simulink library "Lib_Analytic"  (R2019b)
settings: Solver=VariableStepAuto  StartTime=0.0  StopTime=10.0  RelTol=1e-3
undefined symbols (not defined in the file): SJac_Per_M, SNR_DX_M, SNR_IC_M, SNR_Mn_M, SNR_Mx_M
libraries: simulink x2
(part 1 of 2)
settings Model: Creator=sbianco1  LastModifiedBy=sbianco1

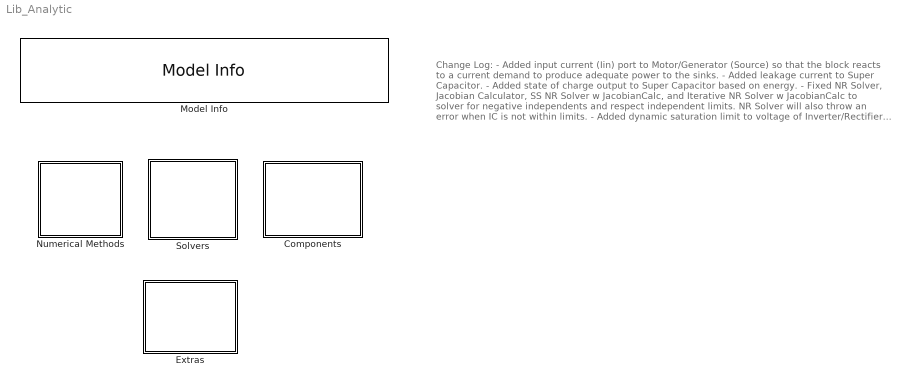
== system Lib_Analytic ==
  note: Change Log:
      | - Added input current (Iin) port to Motor/Generator (Source) so that the block reacts to a current demand to produce adequate power to the sinks.
      | - Added leakage current to Super Capacitor.
      | - Added state of charge output to Super Capacitor based on energy.
      | - Fixed NR Solver, Jacobian Calculator, SS NR Solver w JacobianCalc, and Iterative NR Solver w JacobianCalc to solver for negative independents and respect independent limits. NR Solver will also throw an error when IC is not within limits.
      | - Added dynamic saturation limit to voltage of Inverter/Rectifier (Sink). The back EMF produced by the rotation of the motor limits the voltage output to the motor. It cannot go higher than the input voltage. This limits the speed of the motor.
      | - Added subsystem in multiple blocks inside Components (Analytical) to address calculation problems when Vin = 0.
      | - Created a temperature block.
  Components : Subsystem
  Extras : Subsystem
  Model Info : simulink/Model-Wide Utilities/Model Info  Frame=on  DisplayStringWithTags=|  HorizontalTextAlignment=Left  LeftAlignmentValue=0.02
      | Created by: Santino Bianco and Mark Bell with references from Jeff Chapman.
      | Version: %<ModelVersion>
  Numerical Methods : Subsystem
  Solvers : Subsystem

== system Lib_Analytic/Components ==
  Active Resistor : Subsystem  ClipboardFcn=|  mask(Active Resistor){}
      | Active Resistor
      | Version: %<LibraryVersion>
      mask help: This block changes its resistance (R) based on a power command (Pset) to produce a current demand (Iin).
      settings: AttributesFormatString=|
      | Active Resistor
      | Version: %<LibraryVersion>
  Cable : Subsystem  mask(Cable){R_c=0.2, I_IC=0}
      mask prompts: R_c "R_c - Resistance, Ohm"; I_IC "I_IC - Initial Current, A"
      mask help: This block models a cable with resistive line effects.
      settings: AttributesFormatString=|
      | Cable
      | Version: %<LibraryVersion>
  Current Junction : Subsystem  mask(Current Junction){}
      mask help: This block adds a vector of input currents (I).
      settings: AttributesFormatString=|
      | Current Junction
      | Version: %<LibraryVersion>
      mask DialogControl Control2 Prompt: Note: There is no limit to the number of multiplexed currents.
  DC-DC Converter : Subsystem  mask(DC-DC Converter){X_Vin_VoltageVec_M=[0 100 1000 5000], Y_Iout_CurrentVec_M=[0 10 100 150], T_C_EffArray_M=0.98*ones(4,4)}
      mask prompts: X_Vin_VoltageVec_M "X_Vin_VoltageVec_M - Efficiency Table Voltage Vector (X-axis)(nx1)"; Y_Iout_CurrentVec_M "Y_Iout_CurrentVec_M - Efficiency Table Current Vector (Y-axis)(mx1)"; T_C_EffArray_M "T_C_EffArray_M - Efficiency Table Values (Eff = f(i, V)(nxm)"
      mask help: This block models the power flow through a DC-DC converter using a user specified efficiency table. The output voltage (Vout) can also be set using variable Vset.
      settings: AttributesFormatString=|
      | DC-DC Converter
      | Version: %<LibraryVersion>
  Inverter/Rectifier (Sink) : Subsystem  mask(Inverter/Rectifier - Sink){X_C_VoltageVec_M=[0 100 1000 5000], Y_C_CurrentVec_M=[0 10 100 150], T_C_EffArray_M=.90*ones(4,4), K_e=0.0503}
      mask prompts: X_C_VoltageVec_M "X_C_VoltageVec_M - Efficiency Table Voltage Vector (X-axis)(nx1)"; Y_C_CurrentVec_M "Y_C_CurrentVec_M - Efficiency Table Current Vector (Y-axis)(mx1)"; T_C_EffArray_M "T_C_EffArray_M - Efficiency Table Values (Eff = f(i, V)(nxm)"; K_e "K_e - Back EMF Constant, V/RPM"
      mask help: This block models an inverter/rectifier for use as a power sink. The power through the inverter/rectifier is modified by a user-input efficiency table.
      settings: AttributesFormatString=|
      | Inverter/Rectifier (Sink)
      | Version: %<LibraryVersion>
  Inverter/Rectifier (Source) : Subsystem  mask(Inverter/Rectifier - Source){X_Vout_VoltageVec_M=[0 100 1000 5000], Y_Iin_CurrentVec_M=[0 10 100 150], T_C_EffArray_M=.90*ones(4,4)}
      mask prompts: X_Vout_VoltageVec_M "X_Vout_VoltageVec_M - Efficiency Table Voltage Vector (X-axis)(nx1)"; Y_Iin_CurrentVec_M "Y_Iin_CurrentVec_M - Efficiency Table Current Vector (Y-axis)(mx1)"; T_C_EffArray_M "T_C_EffArray_M - Efficiency Table Values (Eff = f(i, V)(nxm)"
      mask help: This block models an inverter/rectifier for use as a power source. The power through the inverter/rectifier is modified by a user-input efficiency table.
      settings: AttributesFormatString=|
      | Inverter/Rectifier (Source)
      | Version: %<LibraryVersion>
  Mechanical Shaft : Subsystem  mask(Mechanical Shaft){J=0.01, B=0.001, N_IC=0}
      mask prompts: J "J - Inertia, lb-ft-s^2"; B "B - Damping, lb-ft-s"; N_IC "N_IC - Initial Speed, RPM"
      mask help: This block models a mechanical shaft with inertia and damping effects.
      settings: AttributesFormatString=|
      | Mechanical Shaft
      | Version: %<LibraryVersion>
  Motor/Generator (Sink) : Subsystem  mask(Motor/Generator - Sink){X_C_SpeedVec_M=[0 100 1000 5000], Y_C_TorqueVec_M=[0 10 100 150], T_C_EffArray_M=0.99*ones(4,4)}
      mask prompts: X_C_SpeedVec_M "X_C_SpeedVec_M - Efficiency Table Speed Vector (X-axis)(nx1)"; Y_C_TorqueVec_M "Y_C_TorqueVec_M - Efficiency Table Torque Vector (Y-axis)(mx1)"; T_C_EffArray_M "T_C_EffArray_M - Efficiency Table Values (Eff = f(i, V)(nxm)"
      mask help: This block models an motor/generator for use as a power sink. The power through the motor/generator is modified by a user-input efficiency table.
      settings: AttributesFormatString=|
      | Motor/Generator (Sink)
      | Version: %<LibraryVersion>
  Motor/Generator (Source) : Subsystem  mask(Motor/Generator - Source){X_C_SpeedVec_M=[0 100 1000 5000], Y_C_TorqueVec_M=[0 10 100 150], T_C_EffArray_M=0.99*ones(4,4), K_e=0.0503, K_t=0.0503}
      mask prompts: X_C_SpeedVec_M "X_C_SpeedVec_M - Efficiency Table Speed Vector (X-axis)(nx1)"; Y_C_TorqueVec_M "Y_C_TorqueVec_M - Efficiency Table Torque Vector (Y-axis)(mx1)"; T_C_EffArray_M "T_C_EffArray_M - Efficiency Table Values (Eff = f(i, V)(nxm)"; K_e "K_e - Back EMF Constant, V/RPM"; K_t "K_t - Torque Constant, lbf-ft/A"
      mask help: This block models an motor/generator for use as a power source. The power through the motor/generator is modified by a user-input efficiency table.
      settings: AttributesFormatString=|
      | Motor/Generator (Source)
      | Version: %<LibraryVersion>
  Super Capacitor : Subsystem  mask(Super Capacitor){C=130, ESR=0.02, ILeak=0, TSE=69, Iout_IC=0, V_IC=150}
      mask prompts: C "C - Capacitance, H"; ESR "ESR - Equivilent Series Resistance, Ohm"; ILeak "ILeak - Leakage Current per Time Step, A"; TSE "TSE - Max Stored Energy, W-h"; Iout_IC "Iout_IC - Initial Output Current, A"; V_IC "V_IC - Initial Voltage, V"
      mask help: This block models a capacitor with equivilent series resistive (ESR) effects.
      settings: AttributesFormatString=|
      | Super Capacitor
      | Version: %<LibraryVersion>

== system Lib_Analytic/Extras ==
  Exergy : Subsystem  mask(Exergy){m=0, Cp=0}
      mask prompts: m "m - Mass, slug"; Cp "Cp - Specific Heat, Btu/degF"
      mask help: This block calculated the exergy of a component given the component's generated heat, mass, material specific heat, and chnage in ambient temperature from sea level static (SLS).
      settings: AttributesFormatString=|
      | Exergy
      | Version: %<LibraryVersion>
  Temperature : Subsystem  mask(Temperature){m=0, Cp=0}
      mask prompts: m "m - Mass, lbm"; Cp "Cp - Specific Heat, Btu/(lbm-degF)"
      mask help: This block converts a heat output (Heat) from an electrical component to a temperature (Temp) using the ambient temperature (Ambient Temp) and possibly a change in ambient temperature from sea-level static (dTamb) as inputs. A mass in units of pound-mass and a specific heat in units of Btu/(lbm-degF) must be specified.
      settings: AttributesFormatString=|
      | Temperature
      | Version: %<LibraryVersion>
      mask DialogControl Container3 Prompt: Physical Parameters

== system Lib_Analytic/Numerical Methods ==
  Jacobian Calculator : Subsystem  TreatAsAtomicUnit=on  mask(T-MATS: Jacobian Calculator Library Block){N_Per_M=SJac_Per_M}
      mask prompts: N_Per_M "N_Per_M - Perturbations (nxm)"
      mask help:
      | The Jacobian Calculator block calculates the Jabobian of the system by perturbing the system around an initial point and calculating the gradient for each perturbation. This module will run once on start up and then again only if the reset is pressed.
      | Below: n (rows) is the number of times each independent will be perturbed and m (columns) is the number of inputs.
      settings: AttributesFormatString=|
      | Jacobian Calculator
      | Version: %<LibraryVersion>
      mask Help: web(which('NumMthd_TMATS_JC.html'),'-helpbrowser')
  Newton Raphson Solver : Subsystem  TreatAsAtomicUnit=on  mask(T-MATS: Newton Raphson Solver Library Block){NR_IC_M=SNR_IC_M./abs(SNR_IC_M), NR_dx_Lim_M=SNR_DX_M, NR_Mx_Lim_M=SNR_Mx_M./abs(SNR_IC_M), NR_Mn_Lim_M=SNR_Mn_M./abs(SNR_IC_M), BlkNm_M=double(gcb)}
      mask prompts: NR_IC_M "NR_IC_M - Initial Conditions of Newton Raphson (mx1)"; NR_dx_Lim_M "NR_dx_Lim_M - Newton Raphson step size limit (%) (1x1)"; NR_Mx_Lim_M "NR_Mx_Lim_M - Max limit (1x1 or mx1)"; NR_Mn_Lim_M "NR_Mn_Lim_M - Min Limit (1x1 or mx1)"; BlkNm_M "BlkNm_M - Block Name"
      mask help:
      | Newton Raphson Solver:
      |
      | x(n+1) = x(n) - inverse(f'(x(n)))*f(x(n))
      |
      | Note:
      | inverse(f'(x(n))) is an m x m matrix and f(x(n)) is an m x 1 matrix
      | where m is the length of the initial conditions matrix and number of system independents.
      mask init:
      | if isequal(size(NR_Mx_Lim_M),size(NR_IC_M))
      | elseif isequal(size(NR_Mx_Lim_M),size(1))
      | else
      |     warning('NR_Mx_Lim_M must be the same size as NR_IC_M or a constant')
      | end
      | 
      | if isequal(size(NR_Mn_Lim_M),size(NR_IC_M))
      | elseif isequal(size(NR_Mn_Lim_M),size(1))
      | else
      |     warning('NR_Mn_Lim_M must be the same size as NR_IC_M or a constant')
      | end
      settings: AttributesFormatString=|
      | Newton Raphson Solver
      | Version: %<LibraryVersion>
      mask Help: web(which('NumMthd_TMATS_NRS.html'),'-helpbrowser')

== system Lib_Analytic/Solvers ==
  Iterative NR Solver w JacobianCalc : Subsystem  mask(T-MATS: Iterative NR Solver w Jacobian Calc Library Block){SJac_Per_M=0.01*ones(2,2), SNR_IC_M=[-4;1], SNR_DX_M=5, SNR_Mx_M=100000, SNR_Mn_M=-100000, SJacobianAttempts_M=20, Cond_Limits_M=0.0001}
      mask prompts: SJac_Per_M "SJac_Per_M - Jacobian Perturbation size (frac) (nxm)"; SNR_IC_M "SNR_IC_M - Newton Raphson Initial Conditions (mx1)"; SNR_DX_M "SNR_DX_M - Newton Raphson step size limiter (%) (1x1)"; SNR_Mx_M "SNR_Mx_M - Newton Raphson max limit (1x1 or mx1)"; SNR_Mn_M "SNR_Mn_M - Newton Raphson min limit (1x1 or mx1)"; SJacobianAttempts_M "SJacobianAttempts_M - Newton Raphson attempts before the Jacobian recalculation (1x1)"; Cond_Limits_M "Cond_Limits_M - Iteration Conditions Limits (mx1 or 1x1)"
      mask help:
      | The Iterative Newton Raphson Solver with Jacobian Calculator block will
      | supply the inputs to iteratively drive the outputs of a system to zero.
      |
      | This will be performed in three steps.
      | 1) Jabobian calculator sends Perturbations to the plant then calculates the plant
      | Jacboian based on the system response
      | 2) The Newton Raphson will use the inverse of the Jacobian to iteratively step the
      | system toward solution.
      | 3) Once the solution has satisfied the conditions the Newton Raphson is shut off.
      |
      | This module is designed for dynamic systems and should be paired with
      | a "do... while" block in Simulink. The "do...while" block and this module
      | should both be located in the same subsystem as the plant that is to be solved for.
      mask init:
      | if isequal(size(SNR_Mx_M),size(SNR_IC_M))
      | elseif isequal(size(SNR_Mx_M),[1 1])
      | else
      |     disp('NR_Mx_Lim_M must be the same size as NR_IC_M or a constant')
      | end
      | 
      | if isequal(size(SNR_Mn_M),size(SNR_IC_M))
      | elseif isequal(size(SNR_Mn_M),[1 1])
      | else
      |     disp('NR_Mn_Lim_M must be the same size as NR_IC_M or a constant')
      | end
      settings: AttributesFormatString=|
      | Iterative NR Solver w JacobianCalc
      | Version: %<LibraryVersion>
      mask Help: web(which('Solver_TMATS_INRSwJC.html'),'-helpbrowser')
  SS NR Solver w JacobianCalc : Subsystem  mask(T-MATS: SS NR Solver w Jacobian Calc Library Block){SJac_Per_M=0.01*ones(2,2), SNR_IC_M=[-4;5], SNR_DX_M=5, SNR_Mx_M=100000, SNR_Mn_M=-100000, SJacobianAttempts_M=20, Cond_Limits_M=0.0001}
      mask prompts: SJac_Per_M "SJac_Per_M - Jacobian Perturbation size (frac)(nxm)"; SNR_IC_M "SNR_IC_M - Newton Raphson Initial Conditions (mx1)"; SNR_DX_M "SNR_DX_M - Newton Raphson step size limit (%) (1x1)"; SNR_Mx_M "SNR_Mx_M - Newton Raphson max limit (1x1 or mx1)"; SNR_Mn_M "SNR_Mn_M - Newton Raphson min limit (1x1 or mx1)"; SJacobianAttempts_M "SJacobianAttempts_M - Newton Raphson attempts before the Jacobian recalculation (1x1)"; Cond_Limits_M "Cond_Limits_M - Iteration Conditions Limits (mx1 or 1x1)"
      mask help:
      | The Steady State Newton Raphson Solver with Jacobian Calculator block will
      | supply the inputs to iteratively drive the outputs of a system to zero.
      |
      | This will be performed in three steps.
      | 1) Jabobian calculator sends Perturbations to the plant then calculates the plant
      | Jacboian based on the system response
      | 2) The Newton Raphson will use the inverse of the Jacobian to iteratively step the
      | system toward solution.
      | 3) Once the solution has satisfied the conditions the Newton Raphson is shut off.
      |
      | Simulation run time length should be selected as to give the Newton Raphson solver adequate time to develop a solution.
      mask init: same as Lib_Analytic/Solvers/Iterative NR Solver w JacobianCalc
      settings: AttributesFormatString=|
      | SS NR Solver w JacobianCalc
      | Version: %<LibraryVersion>
      mask Help: web(which('Solver_TMATS_SSNRwJC.html'),'-helpbrowser')

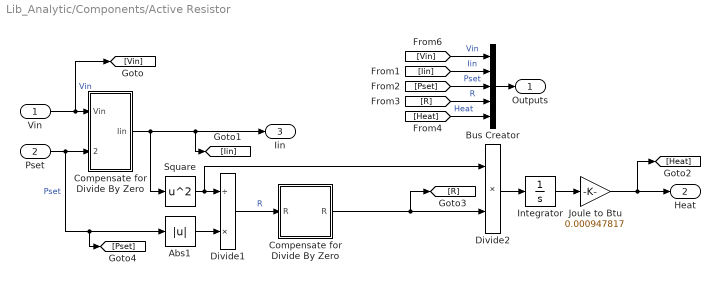
== system Lib_Analytic/Components/Active Resistor ==
  Vin : Inport
  "Pset " : Inport  Port=2
  Abs1 : Abs
  Bus Creator : BusCreator  Inputs=5
  Compensate for Divide By Zero : Subsystem
  "Compensate for Divide By Zero " : Subsystem
  Divide1 : Product  Inputs=/*
  Divide2 : Product  Inputs=**
  Integrator : Integrator
  Joule to Btu : Gain  Gain=0.000947817
  Square : Math  Operator=square  SignedPower=off  SaturateOnIntegerOverflow=on
  Outputs : Outport
  Heat : Outport  Port=2
  Iin : Outport  Port=3
  wires:
  Bus Creator/1 -> Outputs/1
  Divide1/1 -> Compensate for Divide By Zero/1(R)  "R"
  Square/1 -> Divide2/1, Divide1/1
  "Pset "/1 -> "Compensate for Divide By Zero "/2(Pset), [Pset], Abs1/1  "Pset"
  Vin/1 -> [Vin], "Compensate for Divide By Zero "/1(Vin)  "Vin"
  Divide2/1 -> Integrator/1
  Integrator/1 -> Joule to Btu/1
  Joule to Btu/1 -> [Heat], Heat/1
  [Vin] -> Bus Creator/1  "Vin"
  [Iin] -> Bus Creator/2  "Iin"
  [Pset] -> Bus Creator/3  "Pset"
  [R] -> Bus Creator/4  "R"
  [Heat] -> Bus Creator/5  "Heat"
  Abs1/1 -> Divide1/2
  Compensate for Divide By Zero/1("R ") -> [R], Divide2/2
  "Compensate for Divide By Zero "/1(Iin) -> [Iin], Iin/1, Square/1

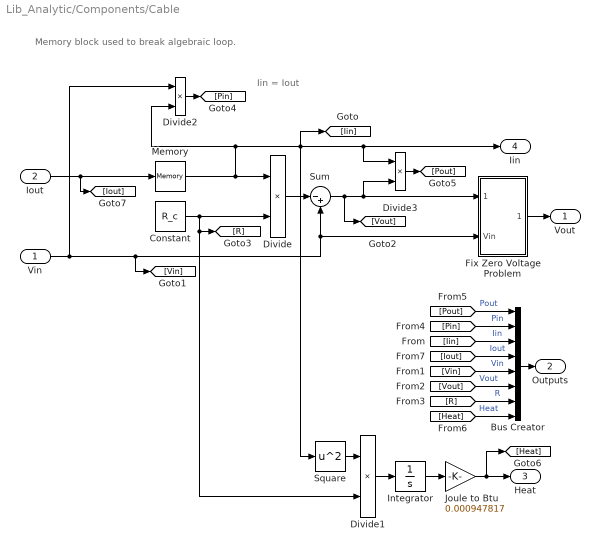
== system Lib_Analytic/Components/Cable ==
  note: Iin = Iout
  note: Memory block used to break algebraic loop.
  Vin : Inport
  Iout : Inport  Port=2
  Bus Creator : BusCreator  Inputs=8
  Constant : Constant  Value=R_c
  Divide{,1..3} (4 alike) : Product  Inputs=**
  Fix Zero Voltage Problem : Subsystem
  Integrator : Integrator
  Joule to Btu : Gain  Gain=0.000947817
  Memory : Memory  InitialCondition=I_IC
  Square : Math  Operator=square  SignedPower=off  SaturateOnIntegerOverflow=on
  Sum : Sum  Inputs=|-+
  Vout : Outport
  Outputs : Outport  Port=2
  Heat : Outport  Port=3
  Iin : Outport  Port=4
  wires:
  Divide/1 -> Sum/1
  Vin/1 -> Divide2/1, Sum/2, Fix Zero Voltage Problem/2(Vin), [Vin]
  Sum/1 -> [Vout], Fix Zero Voltage Problem/1("Vout "), Divide3/2
  Memory/1 -> Square/1, Divide3/1, Iin/1, [Iin], Divide2/2, Divide/1
  Iout/1 -> [Iout], Memory/1
  [Iin] -> Bus Creator/3  "Iin"
  [Vout] -> Bus Creator/6  "Vout"
  [Vin] -> Bus Creator/5  "Vin"
  Bus Creator/1 -> Outputs/1
  [R] -> Bus Creator/7  "R"
  Constant/1 -> Divide1/2, [R], Divide/2
  Square/1 -> Divide1/1
  Divide1/1 -> Integrator/1
  Joule to Btu/1 -> [Heat], Heat/1
  Integrator/1 -> Joule to Btu/1
  [Pin] -> Bus Creator/2  "Pin"
  [Pout] -> Bus Creator/1  "Pout"
  Divide2/1 -> [Pin]
  Divide3/1 -> [Pout]
  [Heat] -> Bus Creator/8  "Heat"
  Fix Zero Voltage Problem/1(Vout) -> Vout/1
  [Iout] -> Bus Creator/4  "Iout"

== system Lib_Analytic/Components/Current Junction ==
  I : Inport
  Sum of Elements : Sum  Inputs=+
  Isum : Outport
  wires:
  I/1 -> Sum of Elements/1
  Sum of Elements/1 -> Isum/1

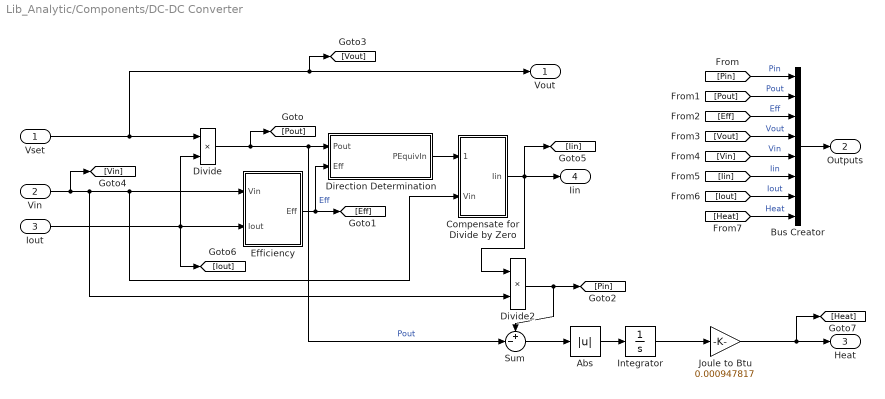
== system Lib_Analytic/Components/DC-DC Converter ==
  Vset : Inport
  Vin : Inport  Port=2
  Iout : Inport  Port=3
  Abs : Abs
  Bus Creator : BusCreator  Inputs=8
  Compensate for Divide by Zero : Subsystem
  Direction Determination : Subsystem
  Divide : Product  Inputs=**
  Divide2 : Product  Inputs=**
  Efficiency : Subsystem
  Integrator : Integrator
  Joule to Btu : Gain  Gain=0.000947817
  Sum : Sum  Inputs=+-|
  Vout : Outport
  Outputs : Outport  Port=2
  Heat : Outport  Port=3
  Iin : Outport  Port=4
  wires:
  Vset/1 -> [Vout], Vout/1, Divide/1
  Joule to Btu/1 -> [Heat], Heat/1
  Vin/1 -> [Vin], Divide2/2, Compensate for Divide by Zero/2(Vin), Efficiency/1(Vin)
  Compensate for Divide by Zero/1(Iin) -> [Iin], Divide2/1, Iin/1
  Direction Determination/1(PEquivIn) -> Compensate for Divide by Zero/1(PEquivIn)
  Efficiency/1(Eff) -> Direction Determination/2(Eff), [Eff]  "Eff"
  Divide/1 -> Sum/2, Direction Determination/1(Pout), [Pout]  "Pout"
  Bus Creator/1 -> Outputs/1
  Divide2/1 -> [Pin], Sum/1
  [Pin] -> Bus Creator/1  "Pin"
  [Pout] -> Bus Creator/2  "Pout"
  [Eff] -> Bus Creator/3  "Eff"
  [Vout] -> Bus Creator/4  "Vout"
  [Vin] -> Bus Creator/5  "Vin"
  [Iin] -> Bus Creator/6  "Iin"
  Iout/1 -> Divide/2, [Iout], Efficiency/2(Iout)
  [Iout] -> Bus Creator/7  "Iout"
  [Heat] -> Bus Creator/8  "Heat"
  Integrator/1 -> Joule to Btu/1
  Abs/1 -> Integrator/1
  Sum/1 -> Abs/1

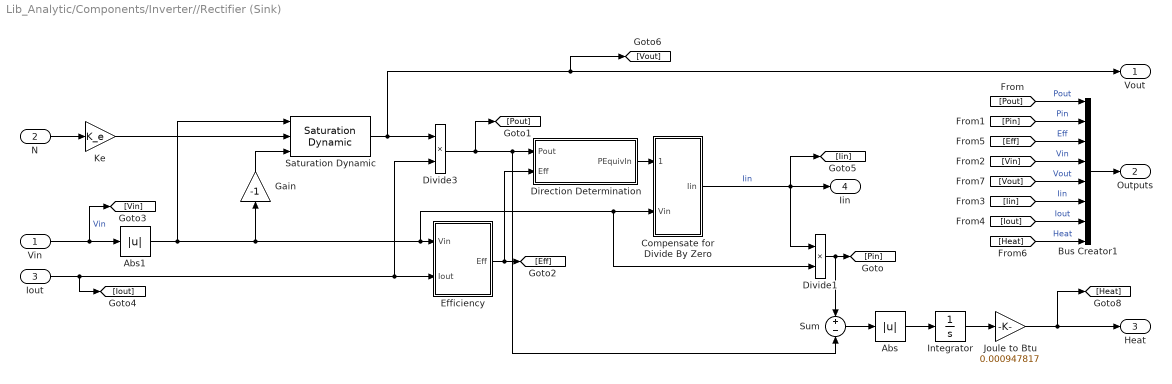
== system Lib_Analytic/Components/Inverter//Rectifier (Sink) ==
  Vin : Inport
  N : Inport  Port=2
  Iout : Inport  Port=3
  Abs : Abs
  Abs1 : Abs
  Bus Creator1 : BusCreator  Inputs=8
  Compensate for Divide By Zero : Subsystem
  Direction Determination : Subsystem
  Divide1 : Product  Inputs=**
  Divide3 : Product  Inputs=**
  Efficiency : Subsystem
  Gain : Gain  Gain=-1
  Integrator : Integrator
  Joule to Btu : Gain  Gain=0.000947817
  Ke : Gain  Gain=K_e
  Saturation Dynamic : simulink/Discontinuities/Saturation Dynamic  OutMin=[]  OutMax=[]  OutDataTypeStr=Inherit: Same as second input  OutDataType=fixdt(1, 16)  OutScaling=2^-10  DoSatur=off
  Sum : Sum  Inputs=+-
  Vout : Outport
  Outputs : Outport  Port=2
  Heat : Outport  Port=3
  Iin : Outport  Port=4
  wires:
  Iout/1 -> [Iout], Efficiency/2(Iout), Divide3/2
  Vin/1 -> [Vin], Abs1/1  "Vin"
  Divide3/1 -> Direction Determination/1(Pout), Sum/2, [Pout]
  Compensate for Divide By Zero/1(Iin) -> [Iin], Divide1/1, Iin/1  "Iin"
  Efficiency/1(Eff) -> [Eff], Direction Determination/2(Eff)
  Ke/1 -> Saturation Dynamic/2
  N/1 -> Ke/1
  [Pin] -> Bus Creator1/2  "Pin"
  [Pout] -> Bus Creator1/1  "Pout"
  [Vin] -> Bus Creator1/4  "Vin"
  [Iin] -> Bus Creator1/6  "Iin"
  Bus Creator1/1 -> Outputs/1
  [Eff] -> Bus Creator1/3  "Eff"
  [Iout] -> Bus Creator1/7  "Iout"
  Direction Determination/1(PEquivIn) -> Compensate for Divide By Zero/1(PEquivIn)
  Divide1/1 -> Sum/1, [Pin]
  [Heat] -> Bus Creator1/8  "Heat"
  [Vout] -> Bus Creator1/5  "Vout"
  Sum/1 -> Abs/1
  Abs/1 -> Integrator/1
  Integrator/1 -> Joule to Btu/1
  Joule to Btu/1 -> [Heat], Heat/1
  Saturation Dynamic/1 -> [Vout], Vout/1, Divide3/1
  Gain/1 -> Saturation Dynamic/3
  Abs1/1 -> Saturation Dynamic/1, Gain/1, Divide1/2, Compensate for Divide By Zero/2(Vin), Efficiency/1(Vin)

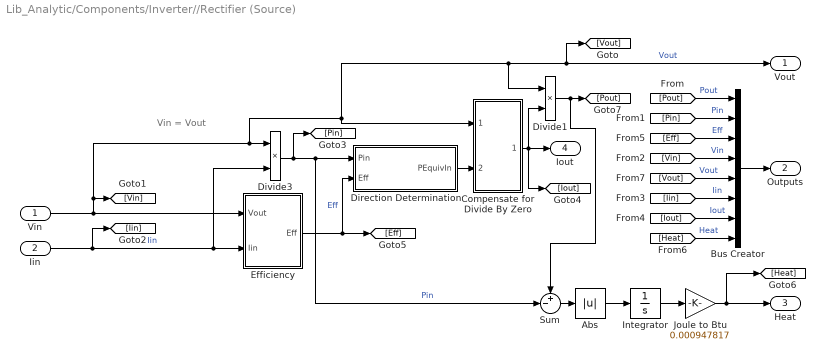
== system Lib_Analytic/Components/Inverter//Rectifier (Source) ==
  note: Vin = Vout
  Vin : Inport
  Iin : Inport  Port=2
  Abs : Abs
  Bus Creator : BusCreator  Inputs=8
  Compensate for Divide By Zero : Subsystem
  Direction Determination : Subsystem
  Divide1 : Product  Inputs=**
  Divide3 : Product  Inputs=**
  Efficiency : Subsystem
  Integrator : Integrator
  Joule to Btu : Gain  Gain=0.000947817
  Sum : Sum  Inputs=+-|
  Vout : Outport
  Outputs : Outport  Port=2
  Heat : Outport  Port=3
  Iout : Outport  Port=4
  wires:
  Vin/1 -> Efficiency/1(Vout), [Vin], Divide3/1, Compensate for Divide By Zero/1(Vout), Divide1/1, [Vout], Vout/1  "Vout"
  Efficiency/1(Eff) -> [Eff], Direction Determination/2(Eff)  "Eff"
  Compensate for Divide By Zero/1(Iout) -> Divide1/2, Iout/1, [Iout]
  Bus Creator/1 -> Outputs/1
  Divide3/1 -> [Pin], Sum/2, Direction Determination/1(Pin)  "Pin"
  Iin/1 -> [Iin], Divide3/2, Efficiency/2(Iin)  "Iin"
  Direction Determination/1(PEquivIn) -> Compensate for Divide By Zero/2(PEquivIn)
  [Pout] -> Bus Creator/1  "Pout"
  [Pin] -> Bus Creator/2  "Pin"
  [Vin] -> Bus Creator/4  "Vin"
  [Iin] -> Bus Creator/6  "Iin"
  [Iout] -> Bus Creator/7  "Iout"
  [Eff] -> Bus Creator/3  "Eff"
  [Heat] -> Bus Creator/8  "Heat"
  Integrator/1 -> Joule to Btu/1
  Sum/1 -> Abs/1
  Abs/1 -> Integrator/1
  Joule to Btu/1 -> [Heat], Heat/1
  Divide1/1 -> Sum/1, [Pout]
  [Vout] -> Bus Creator/5  "Vout"

== system Lib_Analytic/Components/Mechanical Shaft ==
  note: Units
      | J : lb-ft-s^2
      | B : lb-ft-s
  T : Inport
  Abs : Abs
  Bus Creator : BusCreator  Inputs=3
  Gain : Gain  Gain=1/J
  Gain1 : Gain  Gain=B
  Integrator : Integrator  InitialCondition=N_IC*(2*pi/60)
  Joule to Btu : Gain  Gain=0.000947817
  Sum : Sum  Inputs=|+-
  Sum of Elements : Sum  Inputs=+
  lbf-ft to J : Gain  Gain=1.355818
  rad/s to RPM : Gain  Gain=60/(2*pi)
  N : Outport
  Outputs : Outport  Port=2
  Heat : Outport  Port=3
  wires:
  Bus Creator/1 -> Outputs/1
  rad/s to RPM/1 -> [N], N/1
  Sum of Elements/1 -> Sum/1
  Gain/1 -> Integrator/1
  Integrator/1 -> Gain1/1, rad/s to RPM/1
  T/1 -> Sum of Elements/1
  [Tnet] -> Bus Creator/1  "Tnet"
  [N] -> Bus Creator/2  "N"
  [Heat] -> Bus Creator/3  "Heat"
  Joule to Btu/1 -> Heat/1, [Heat]
  Sum/1 -> [Tnet], Gain/1
  Gain1/1 -> lbf-ft to J/1, Sum/2
  Abs/1 -> Joule to Btu/1
  lbf-ft to J/1 -> Abs/1

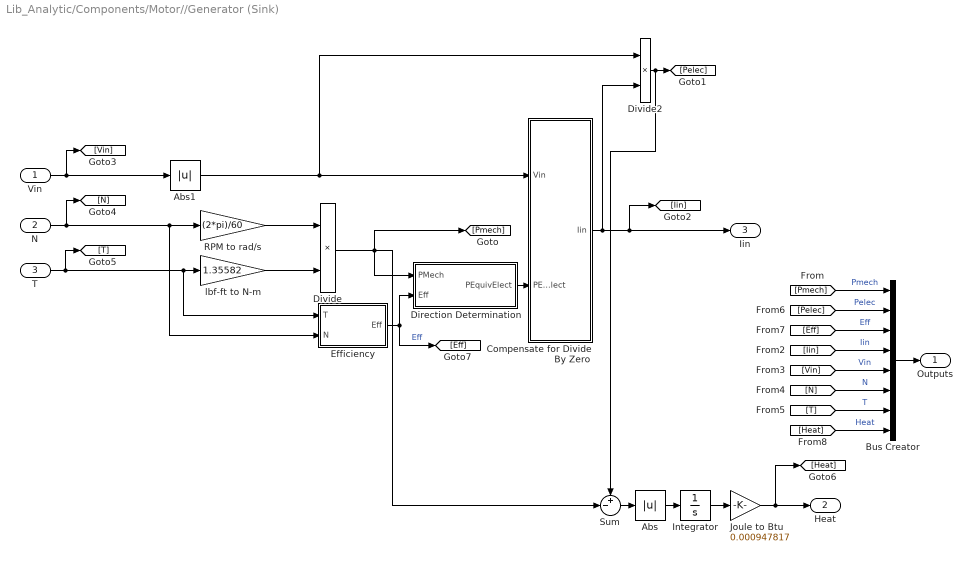
== system Lib_Analytic/Components/Motor//Generator (Sink) ==
  Vin : Inport
  N : Inport  Port=2
  T : Inport  Port=3
  Abs : Abs
  Abs1 : Abs
  Bus Creator : BusCreator  Inputs=8
  Compensate for Divide By Zero : Subsystem
  Direction Determination : Subsystem
  Divide : Product  Inputs=**
  Divide2 : Product  Inputs=**
  Efficiency : Subsystem
  Integrator : Integrator
  Joule to Btu : Gain  Gain=0.000947817
  RPM to rad/s : Gain  Gain=(2*pi)/60
  Sum : Sum  Inputs=+-|
  lbf-ft to N-m : Gain  Gain=1.35582
  Outputs : Outport
  Heat : Outport  Port=2
  Iin : Outport  Port=3
  wires:
  Bus Creator/1 -> Outputs/1
  Efficiency/1(Eff) -> [Eff], Direction Determination/2(Eff)  "Eff"
  Vin/1 -> [Vin], Abs1/1
  lbf-ft to N-m/1 -> Divide/2
  RPM to rad/s/1 -> Divide/1
  T/1 -> Efficiency/1(T), lbf-ft to N-m/1, [T]
  Divide/1 -> [Pmech], Sum/2, Direction Determination/1(PMech)
  [Pmech] -> Bus Creator/1  "Pmech"
  Divide2/1 -> Sum/1, [Pelec]
  [Iin] -> Bus Creator/4  "Iin"
  [Vin] -> Bus Creator/5  "Vin"
  [N] -> Bus Creator/6  "N"
  [T] -> Bus Creator/7  "T"
  [Eff] -> Bus Creator/3  "Eff"
  [Heat] -> Bus Creator/8  "Heat"
  Sum/1 -> Abs/1
  Abs/1 -> Integrator/1
  Integrator/1 -> Joule to Btu/1
  [Pelec] -> Bus Creator/2  "Pelec"
  Joule to Btu/1 -> [Heat], Heat/1
  Compensate for Divide By Zero/1(Iin) -> [Iin], Iin/1, Divide2/2
  Direction Determination/1(PEquivElect) -> Compensate for Divide By Zero/2(PEquivElect)
  Abs1/1 -> Compensate for Divide By Zero/1(Vin), Divide2/1
  N/1 -> RPM to rad/s/1, Efficiency/2(N), [N]

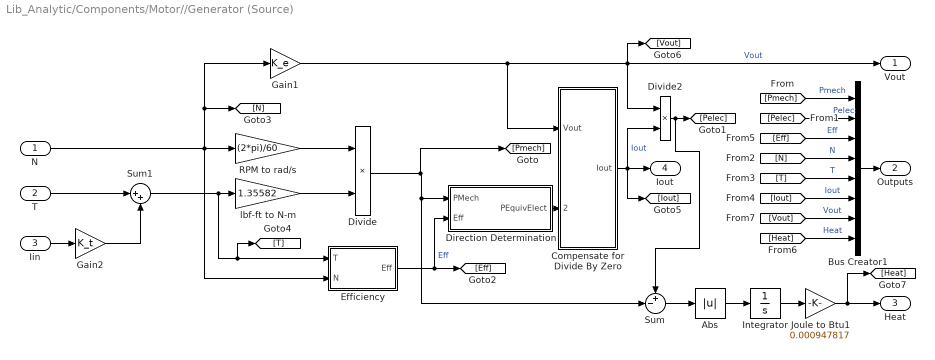
== system Lib_Analytic/Components/Motor//Generator (Source) ==
  N : Inport
  T : Inport  Port=2
  Iin : Inport  Port=3
  Abs : Abs
  Bus Creator1 : BusCreator  Inputs=8
  Compensate for Divide By Zero : Subsystem
  Direction Determination : Subsystem
  Divide : Product  Inputs=**
  Divide2 : Product  Inputs=**
  Efficiency : Subsystem
  Gain1 : Gain  Gain=K_e
  Gain2 : Gain  Gain=K_t
  Integrator : Integrator
  Joule to Btu1 : Gain  Gain=0.000947817
  RPM to rad/s : Gain  Gain=(2*pi)/60
  Sum : Sum  Inputs=+-|
  Sum1 : Sum  Inputs=|++
  lbf-ft to N-m : Gain  Gain=1.35582
  Vout : Outport
  Outputs : Outport  Port=2
  Heat : Outport  Port=3
  Iout : Outport  Port=4
  wires:
  Direction Determination/1(PEquivElect) -> Compensate for Divide By Zero/2(PEquivElect)
  Compensate for Divide By Zero/1(Iout) -> [Iout], Iout/1, Divide2/2  "Iout"
  Efficiency/1(Eff) -> [Eff], Direction Determination/2(Eff)  "Eff"
  lbf-ft to N-m/1 -> Divide/2
  RPM to rad/s/1 -> Divide/1
  Sum1/1 -> [T], Efficiency/1(T), lbf-ft to N-m/1
  N/1 -> [N], Gain1/1, RPM to rad/s/1, Efficiency/2(N)
  Gain1/1 -> Compensate for Divide By Zero/1(Vout), Divide2/1, [Vout], Vout/1  "Vout"
  [Pelec] -> Bus Creator1/2  "Pelec"
  [Heat] -> Bus Creator1/8  "Heat"
  [Pmech] -> Bus Creator1/1  "Pmech"
  [N] -> Bus Creator1/4  "N"
  [T] -> Bus Creator1/5  "T"
  Bus Creator1/1 -> Outputs/1
  [Eff] -> Bus Creator1/3  "Eff"
  [Iout] -> Bus Creator1/6  "Iout"
  Divide/1 -> [Pmech], Sum/2, Direction Determination/1(PMech)
  Divide2/1 -> Sum/1, [Pelec]
  [Vout] -> Bus Creator1/7  "Vout"
  Sum/1 -> Abs/1
  Abs/1 -> Integrator/1
  Integrator/1 -> Joule to Btu1/1
  Joule to Btu1/1 -> [Heat], Heat/1
  T/1 -> Sum1/1
  Iin/1 -> Gain2/1
  Gain2/1 -> Sum1/2

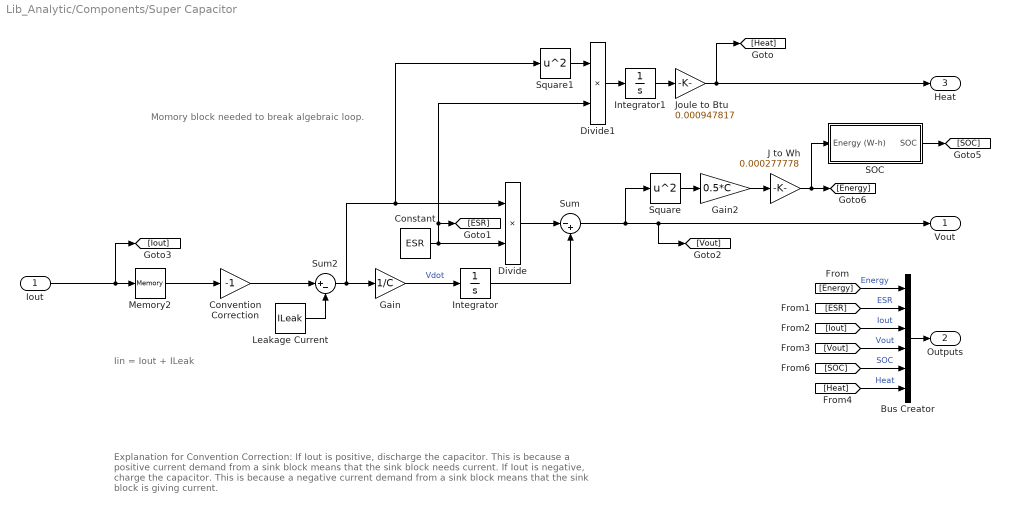
== system Lib_Analytic/Components/Super Capacitor ==
  note: Explanation for Convention Correction:
      | If Iout is positive, discharge the capacitor. This is because a positive current demand from a sink block means that the sink block needs current.
      | If Iout is negative, charge the capacitor. This is because a negative current demand from a sink block means that the sink block is giving current.
  note: Momory block needed to break algebraic loop.
  note: Iin = Iout + ILeak
  "Iout " : Inport
  Bus Creator : BusCreator  Inputs=6
  Constant : Constant  Value=ESR
  Convention Correction : Gain  Gain=-1
  Divide : Product  Inputs=**
  Divide1 : Product  Inputs=**
  Gain : Gain  Gain=1/C
  Gain2 : Gain  Gain=0.5*C
  Integrator : Integrator  InitialCondition=V_IC
  Integrator1 : Integrator
  J to Wh : Gain  Gain=0.000277778
  Joule to Btu : Gain  Gain=0.000947817
  Leakage Current : Constant  Value=ILeak
  Memory2 : Memory  InitialCondition=Iout_IC
  SOC : Subsystem
  Square : Math  Operator=square  SignedPower=off  SaturateOnIntegerOverflow=on
  Square1 : Math  Operator=square  SignedPower=off  SaturateOnIntegerOverflow=on
  Sum : Sum  Inputs=|-+
  Sum2 : Sum  Inputs=|+-
  Vout : Outport
  Outputs : Outport  Port=2
  Heat : Outport  Port=3
  wires:
  Memory2/1 -> Convention Correction/1
  SOC/1(SOC) -> [SOC]
  [SOC] -> Bus Creator/5  "SOC"
  J to Wh/1 -> [Energy], SOC/1(Energy (W-h))
  Leakage Current/1 -> Sum2/2
  Joule to Btu/1 -> [Heat], Heat/1
  [Heat] -> Bus Creator/6  "Heat"
  "Iout "/1 -> [Iout], Memory2/1
  Integrator1/1 -> Joule to Btu/1
  Divide1/1 -> Integrator1/1
  Square1/1 -> Divide1/1
  Bus Creator/1 -> Outputs/1
  [Vout] -> Bus Creator/4  "Vout"
  [Iout] -> Bus Creator/3  "Iout"
  [ESR] -> Bus Creator/2  "ESR"
  [Energy] -> Bus Creator/1  "Energy"
  Gain/1 -> Integrator/1  "Vdot"
  Square/1 -> Gain2/1
  Gain2/1 -> J to Wh/1
  Convention Correction/1 -> Sum2/1
  Integrator/1 -> Sum/2
  Divide/1 -> Sum/1
  Sum/1 -> Square/1, Vout/1, [Vout]
  Constant/1 -> [ESR], Divide1/2, Divide/2
  Sum2/1 -> Square1/1, Divide/1, Gain/1

== system Lib_Analytic/Extras/Exergy ==
  note: X = Q - m*Cp*dTamb
  Heat : Inport
  dTamb : Inport  Port=2
  Divide : Product  Inputs=***
  Mass (slug) : Constant  Value=m
  Specific Heat (Btu/degF) : Constant  Value=Cp
  Sum : Sum  Inputs=|+-
  Exergy : Outport
  wires:
  Heat/1 -> Sum/1
  dTamb/1 -> Divide/1
  Mass (slug)/1 -> Divide/2
  Specific Heat (Btu/degF)/1 -> Divide/3
  Divide/1 -> Sum/2
  Sum/1 -> Exergy/1

== system Lib_Analytic/Extras/Temperature ==
  Heat : Inport
  dTamb : Inport  Port=2
  Tamb : Inport  Port=3
  Divide : Product  Inputs=*//
  Mass (lbm) : Constant  Value=m
  Specific Heat (Btu/(lbm-degF)) : Constant  Value=Cp
  Sum : Sum  Inputs=|++
  Sum1 : Sum  Inputs=|++
  Temp : Outport
  wires:
  Heat/1 -> Divide/1
  Divide/1 -> Sum/1
  Sum1/1 -> Sum/2
  Sum/1 -> Temp/1
  Mass (lbm)/1 -> Divide/2
  Specific Heat (Btu/(lbm-degF))/1 -> Divide/3
  Tamb/1 -> Sum1/2
  dTamb/1 -> Sum1/1

== system Lib_Analytic/Numerical Methods/Jacobian Calculator ==
  Reset : Inport  PortDimensions=1
  f(x_p) : Inport  Port=2  PortDimensions=size(N_Per_M,2)
  Xo : Inport  Port=3  PortDimensions=size(N_Per_M,2)
  Constant2 : Constant  Value=N_Per_M
  Counter : Subsystem  mask{N_Ind_M=prod(size(N_Per_M))}
      mask prompts: N_Ind_M "number of independents, N_Ind_M"
  Jacobian : Subsystem
  Terminator : Terminator
  J : Outport  PortDimensions=[size(N_Per_M,2), size(N_Per_M,2)]
  x_p : Outport  Port=2  PortDimensions=size(N_Per_M,2)
  Iteration : Outport  Port=3  PortDimensions=1
  Active : Outport  Port=4  PortDimensions=1
  inv(J) : Outport  Port=5  PortDimensions=[size(N_Per_M,2), size(N_Per_M,2)]
  JacFailed : Outport  Port=6  PortDimensions=1
  wires:
  Jacobian/5(JacFailed) -> JacFailed/1
  Jacobian/4(y_State) -> Terminator/1
  Jacobian/3(J) -> J/1
  Jacobian/2(Inv(J)) -> inv(J)/1
  Counter/2(Iteration) -> Jacobian/1(Iteration), Iteration/1
  Xo/1 -> Jacobian/4(Xo)
  Counter/1(Enable) -> Jacobian/Enable, Active/1
  Reset/1 -> Counter/1(Reset)
  Jacobian/1(x_p) -> x_p/1
  Constant2/1 -> Jacobian/2(Per)
  f(x_p)/1 -> Jacobian/3(f(x_p))

== system Lib_Analytic/Numerical Methods/Newton Raphson Solver ==
  Enable : Inport  PortDimensions=1
  inv(f'(x(n))) : Inport  Port=2  PortDimensions=[length(NR_IC_M),length(NR_IC_M)]
  f(x(n)) : Inport  Port=3  PortDimensions=length(NR_IC_M)
  NR Update : Subsystem
  Switch : Switch  Criteria=u2 > Threshold
  Unit Delay : UnitDelay  InitialCondition=NR_IC_M  SampleTime=-1  HasFrameUpgradeWarning=on
  x(n) : Outport  PortDimensions=length(NR_IC_M)
  x(n+1) : Outport  Port=2  PortDimensions=length(NR_IC_M)
  wires:
  NR Update/1(x(n+1)) -> Switch/1
  inv(f'(x(n)))/1 -> NR Update/2(inv(J))
  f(x(n))/1 -> NR Update/1(f(x))
  Switch/1 -> x(n+1)/1, Unit Delay/1
  Enable/1 -> NR Update/Enable, Switch/2
  Unit Delay/1 -> NR Update/3(x(n)), Switch/3, x(n)/1

== system Lib_Analytic/Solvers/Iterative NR Solver w JacobianCalc ==
  Iterations : Inport  PortDimensions=1
  Enable : Inport  Port=2  PortDimensions=1
  f(x) : Inport  Port=3  PortDimensions=length(SNR_IC_M)
  Bus Creator : BusCreator  Inputs=2
  JC w Reset : Subsystem
  Logical Operator : Logic  AllPortsSameDT=off  OutDataTypeStr=boolean
  NRwCond : Subsystem
  do_while Condition : Outport  PortDimensions=1
  X : Outport  Port=2  PortDimensions=length(SNR_IC_M)
  S_Data : Outport  Port=3
  wires:
  f(x)/1 -> NRwCond/1(f(x)), JC w Reset/1(f(x))
  NRwCond/1(CCnd) -> Logical Operator/2
  Iterations/1 -> JC w Reset/2(Iter)
  NRwCond/2(x(n+1)) -> JC w Reset/3(x(n+1))
  JC w Reset/1(J) -> Bus Creator/1
  JC w Reset/3(X_out) -> X/1
  JC w Reset/4(JC_Active) -> NRwCond/2(JC_Active)
  JC w Reset/5(inv(J)) -> NRwCond/3(inv(f'(x)))
  Enable/1 -> JC w Reset/Enable, NRwCond/Enable, Logical Operator/1
  Logical Operator/1 -> do_while Condition/1
  Bus Creator/1 -> S_Data/1
  JC w Reset/2(JacFailed) -> Bus Creator/2

== system Lib_Analytic/Solvers/SS NR Solver w JacobianCalc ==
  Enable : Inport  PortDimensions=1
  f(x) : Inport  Port=2  PortDimensions=length(SNR_IC_M)
  Bus Creator : BusCreator  Inputs=3
  JacCalc w Reset : Subsystem  TreatAsAtomicUnit=on
  NewRaph w Cond : Subsystem  TreatAsAtomicUnit=on
  X : Outport  PortDimensions=length(SNR_IC_M)
  S_Data : Outport  Port=2  PortDimensions={1,[length(SNR_IC_M),length(SNR_IC_M)]}
  wires:
  JacCalc w Reset/1(X_out) -> X/1
  JacCalc w Reset/2(JC_Active) -> NewRaph w Cond/2(JC_Active)
  JacCalc w Reset/3(inv(J)) -> NewRaph w Cond/3(inv(f'x(n)))
  JacCalc w Reset/4(J) -> [J]
  NewRaph w Cond/2(CCnd) -> JacCalc w Reset/2(CCnd)
  f(x)/1 -> NewRaph w Cond/1(f(x(n))), JacCalc w Reset/1(f(x))
  NewRaph w Cond/3(x(n+1)) -> JacCalc w Reset/3(x(n+1))
  NewRaph w Cond/1(Converged) -> Bus Creator/1  "Converged"
  Enable/1 -> NewRaph w Cond/Enable, JacCalc w Reset/Enable
  JacCalc w Reset/5(JacFailed) -> [JacFailed]
  Bus Creator/1 -> S_Data/1
  [J] -> Bus Creator/2  "J"
  [JacFailed] -> Bus Creator/3  "JacFailed"

== system Lib_Analytic/Components/Active Resistor/Compensate for Divide By Zero ==
  note: If R is INF (Vin = 0 and Pset ~=0), then set R to zero.
      | If R is NAN (Vin = 0 and Pset = 0), then set R to zero.
      | If R is a value, then use calculated R value.
  R : Inport
  Constant : Constant  Value=0
  IsNaN : RelationalOperator  Operator=isInf  OutDataTypeStr=boolean  RndMeth=Simplest
  IsNaN1 : RelationalOperator  Operator=isNaN  OutDataTypeStr=boolean  RndMeth=Simplest
  Logical Operator : Logic  Operator=OR  AllPortsSameDT=off  OutDataTypeStr=boolean
  Switch : Switch  Criteria=u2 > Threshold
  "R " : Outport
  wires:
  R/1 -> Switch/3, IsNaN1/1, IsNaN/1
  Constant/1 -> Switch/1
  IsNaN/1 -> Logical Operator/1
  Logical Operator/1 -> Switch/2
  IsNaN1/1 -> Logical Operator/2
  Switch/1 -> "R "/1

== system Lib_Analytic/Components/Active Resistor/Compensate for Divide By Zero  ==
  note: If Vin is not zero, then use calculated Iin.
      | If Vin is zero, set Iin to zero.
  Vin : Inport
  Pset : Inport  Port=2
  Constant : Constant  Value=0
  Divide : Product  Inputs=/*
  Switch : Switch  Criteria=u2 ~= 0
  Iin : Outport
  wires:
  Vin/1 -> Switch/2, Divide/1
  Pset/1 -> Divide/2
  Divide/1 -> Switch/1  "Iin"
  Switch/1 -> Iin/1
  Constant/1 -> Switch/3

== system Lib_Analytic/Components/Cable/Fix Zero Voltage Problem ==
  note: If Vin is not equal to zero, pass Vout.
      | If Vin is equal to zero, set Vout to zero. This has to be done because a Vin of 0 would take an efficiency hit and produce a negative Vout.
      | In reality, a zero voltage does not take an efficiency hit.
  "Vout " : Inport
  Vin : Inport  Port=2
  Constant : Constant  Value=0
  Switch : Switch  Criteria=u2 ~= 0
  Vout : Outport
  wires:
  Vin/1 -> Switch/2
  "Vout "/1 -> Switch/1
  Constant/1 -> Switch/3
  Switch/1 -> Vout/1

== system Lib_Analytic/Components/DC-DC Converter/Compensate for Divide by Zero ==
  note: If Vin is not equal to zero, use its value.
      | If Vin is equal to zero, it will calculate a nan value for Iin. Set Iin to zero.
  PEquivIn : Inport
  Vin : Inport  Port=2
  Constant : Constant  Value=0
  Divide : Product  Inputs=/*
  Switch : Switch  Criteria=u2 ~= 0
  Iin : Outport
  wires:
  Switch/1 -> Iin/1
  Divide/1 -> Switch/1
  PEquivIn/1 -> Divide/2
  Vin/1 -> Switch/2, Divide/1
  Constant/1 -> Switch/3

== system Lib_Analytic/Components/DC-DC Converter/Direction Determination ==
  Pout : Inport
  Eff : Inport  Port=2
  Divide : Product  Inputs=/*
  Divide1 : Product  Inputs=**
  Switch : Switch  Criteria=u2 > Threshold
  PEquivIn : Outport
  wires:
  Pout/1 -> Divide1/1, Divide/2, Switch/2
  Divide/1 -> Switch/1
  Divide1/1 -> Switch/3
  Eff/1 -> Divide/1, Divide1/2
  Switch/1 -> PEquivIn/1

== system Lib_Analytic/Components/DC-DC Converter/Efficiency ==
  Vin : Inport
  Iout : Inport  Port=2
  0.1 to 1 : Saturate  UpperLimit=1  LowerLimit=0.1
  2-D Lookup Table : Lookup_n-D  BreakpointsForDimension1=X_Vin_VoltageVec_M  BreakpointsForDimension2=Y_Iout_CurrentVec_M  Table=T_C_EffArray_M  InternalRulePriority=Speed  RndMeth=Simplest  InputSameDT=on
  Abs : Abs
  Abs1 : Abs
  Eff : Outport
  wires:
  Vin/1 -> Abs/1
  Abs/1 -> 2-D Lookup Table/1
  Abs1/1 -> 2-D Lookup Table/2
  Iout/1 -> Abs1/1
  2-D Lookup Table/1 -> 0.1 to 1/1
  0.1 to 1/1 -> Eff/1

== system Lib_Analytic/Components/Inverter//Rectifier (Sink)/Compensate for Divide By Zero ==
  note: If Vin is not equal to zero, use its value.
      | If Vin is equal to zero, it will calculate a nan value for Iin. Set Iin to zero.
  PEquivIn : Inport
  Vin : Inport  Port=2
  Constant : Constant  Value=0
  Divide1 : Product  Inputs=/*
  Switch : Switch  Criteria=u2 ~= 0
  Iin : Outport
  wires:
  Switch/1 -> Iin/1
  Constant/1 -> Switch/3
  Divide1/1 -> Switch/1  "Iin"
  PEquivIn/1 -> Divide1/2
  Vin/1 -> Switch/2, Divide1/1

== system Lib_Analytic/Components/Inverter//Rectifier (Sink)/Direction Determination ==
  Pout : Inport
  Eff : Inport  Port=2
  Divide : Product  Inputs=/*
  Divide1 : Product  Inputs=**
  Switch : Switch  Criteria=u2 > Threshold
  PEquivIn : Outport
  wires:
  Switch/1 -> PEquivIn/1
  Eff/1 -> Divide1/2, Divide/1
  Divide1/1 -> Switch/3
  Divide/1 -> Switch/1
  Pout/1 -> Switch/2, Divide/2, Divide1/1

== system Lib_Analytic/Components/Inverter//Rectifier (Sink)/Efficiency ==
  Vin : Inport
  Iout : Inport  Port=2
  0.1 to 1 : Saturate  UpperLimit=1  LowerLimit=0.1
  2-D Lookup Table : Lookup_n-D  BreakpointsForDimension1=X_C_VoltageVec_M  BreakpointsForDimension2=Y_C_CurrentVec_M  Table=T_C_EffArray_M  InternalRulePriority=Speed  RndMeth=Simplest  InputSameDT=on
  Abs : Abs
  Abs1 : Abs
  Eff : Outport
  wires:
  0.1 to 1/1 -> Eff/1
  2-D Lookup Table/1 -> 0.1 to 1/1
  Iout/1 -> Abs1/1
  Abs1/1 -> 2-D Lookup Table/2
  Abs/1 -> 2-D Lookup Table/1
  Vin/1 -> Abs/1

== system Lib_Analytic/Components/Inverter//Rectifier (Source)/Compensate for Divide By Zero ==
  note: If Vout is not equal to zero, use its value.
      | If Vout is equal to zero, it will calculate a nan value for Iout. Set Iout to zero.
  Vout : Inport
  PEquivIn : Inport  Port=2
  Constant : Constant  Value=0
  Divide1 : Product  Inputs=/*
  Switch : Switch  Criteria=u2 ~= 0
  Iout : Outport
  wires:
  Switch/1 -> Iout/1
  Constant/1 -> Switch/3
  Divide1/1 -> Switch/1  "Iin"
  PEquivIn/1 -> Divide1/2
  Vout/1 -> Switch/2, Divide1/1

== system Lib_Analytic/Components/Inverter//Rectifier (Source)/Direction Determination ==
  Pin : Inport
  Eff : Inport  Port=2
  Divide2 : Product  Inputs=*/
  Divide3 : Product  Inputs=**
  Switch : Switch  Criteria=u2 > Threshold
  PEquivIn : Outport
  wires:
  Pin/1 -> Switch/2, Divide2/1, Divide3/2
  Divide3/1 -> Switch/1
  Divide2/1 -> Switch/3
  Eff/1 -> Divide2/2, Divide3/1
  Switch/1 -> PEquivIn/1

== system Lib_Analytic/Components/Inverter//Rectifier (Source)/Efficiency ==
  Vout : Inport
  Iin : Inport  Port=2
  0.1 to 1 : Saturate  UpperLimit=1  LowerLimit=0.1
  2-D Lookup Table : Lookup_n-D  BreakpointsForDimension1=X_Vout_VoltageVec_M  BreakpointsForDimension2=Y_Iin_CurrentVec_M  Table=T_C_EffArray_M  InternalRulePriority=Speed  RndMeth=Simplest  InputSameDT=on
  Abs : Abs
  Abs1 : Abs
  Eff : Outport
  wires:
  Vout/1 -> Abs/1
  Abs/1 -> 2-D Lookup Table/1
  Abs1/1 -> 2-D Lookup Table/2
  Iin/1 -> Abs1/1
  2-D Lookup Table/1 -> 0.1 to 1/1
  0.1 to 1/1 -> Eff/1

== system Lib_Analytic/Components/Motor//Generator (Sink)/Compensate for Divide By Zero ==
  note: If Vin is not equal to zero, use its value.
      | If Vin is equal to zero, it will calculate a nan value for Iin. Set Iin to zero.
  Vin : Inport
  PEquivElect : Inport  Port=2
  Constant : Constant  Value=0
  Divide1 : Product  Inputs=/*
  Switch : Switch  Criteria=u2 ~= 0
  Iin : Outport
  wires:
  Divide1/1 -> Switch/1  "Iin"
  Vin/1 -> Switch/2, Divide1/1
  PEquivElect/1 -> Divide1/2
  Switch/1 -> Iin/1
  Constant/1 -> Switch/3

== system Lib_Analytic/Components/Motor//Generator (Sink)/Direction Determination ==
  PMech : Inport
  Eff : Inport  Port=2
  Divide : Product  Inputs=/*
  Divide1 : Product  Inputs=**
  Switch : Switch  Criteria=u2 > Threshold
  PEquivElect : Outport
  wires:
  Switch/1 -> PEquivElect/1
  Eff/1 -> Divide1/2, Divide/1
  Divide1/1 -> Switch/3
  Divide/1 -> Switch/1
  PMech/1 -> Switch/2, Divide/2, Divide1/1

== system Lib_Analytic/Components/Motor//Generator (Sink)/Efficiency ==
  T : Inport
  N : Inport  Port=2
  0.1 to 1 : Saturate  UpperLimit=1  LowerLimit=0.1
  2-D Lookup Table : Lookup_n-D  BreakpointsForDimension1=X_C_SpeedVec_M  BreakpointsForDimension2=Y_C_TorqueVec_M  Table=T_C_EffArray_M  InternalRulePriority=Speed  RndMeth=Simplest  InputSameDT=on
  Abs : Abs
  Abs1 : Abs
  Eff : Outport
  wires:
  0.1 to 1/1 -> Eff/1
  2-D Lookup Table/1 -> 0.1 to 1/1
  N/1 -> Abs1/1
  Abs1/1 -> 2-D Lookup Table/2
  Abs/1 -> 2-D Lookup Table/1
  T/1 -> Abs/1

== system Lib_Analytic/Components/Motor//Generator (Source)/Compensate for Divide By Zero ==
  note: If Vout is not equal to zero, use its value.
      | If Vout is equal to zero, it will calculate a nan value for Iout. Set Iout to zero.
  Vout : Inport
  PEquivElect : Inport  Port=2
  Constant : Constant  Value=0
  Divide1 : Product  Inputs=/*
  Switch : Switch  Criteria=u2 ~= 0
  Iout : Outport
  wires:
  PEquivElect/1 -> Divide1/2
  Divide1/1 -> Switch/1  "Iin"
  Constant/1 -> Switch/3
  Vout/1 -> Switch/2, Divide1/1
  Switch/1 -> Iout/1

== system Lib_Analytic/Components/Motor//Generator (Source)/Direction Determination ==
  PMech : Inport
  Eff : Inport  Port=2
  Divide2 : Product  Inputs=*/
  Divide3 : Product  Inputs=**
  Switch : Switch  Criteria=u2 > Threshold
  PEquivElect : Outport
  wires:
  Switch/1 -> PEquivElect/1
  Eff/1 -> Divide2/2, Divide3/1
  Divide2/1 -> Switch/3
  Divide3/1 -> Switch/1
  PMech/1 -> Divide2/1, Divide3/2, Switch/2

== system Lib_Analytic/Components/Motor//Generator (Source)/Efficiency ==
  T : Inport
  N : Inport  Port=2
  0.1 to 1 : Saturate  UpperLimit=1  LowerLimit=0.1
  2-D Lookup Table : Lookup_n-D  BreakpointsForDimension1=X_C_SpeedVec_M  BreakpointsForDimension2=Y_C_TorqueVec_M  Table=T_C_EffArray_M  InternalRulePriority=Speed  RndMeth=Simplest  InputSameDT=on
  Abs : Abs
  Abs1 : Abs
  Eff : Outport
  wires:
  0.1 to 1/1 -> Eff/1
  2-D Lookup Table/1 -> 0.1 to 1/1
  N/1 -> Abs1/1
  Abs1/1 -> 2-D Lookup Table/2
  Abs/1 -> 2-D Lookup Table/1
  T/1 -> Abs/1

== system Lib_Analytic/Components/Super Capacitor/SOC ==
  Energy (W-h) : Inport
  Divide : Product  Inputs=*/
  Gain : Gain  Gain=100
  Total Stored Energy (W-h) : Constant  Value=TSE
  SOC : Outport
  wires:
  Gain/1 -> SOC/1
  Divide/1 -> Gain/1
  Total Stored Energy (W-h)/1 -> Divide/2
  Energy (W-h)/1 -> Divide/1

== system Lib_Analytic/Numerical Methods/Jacobian Calculator/Counter ==
  Reset : Inport
  Constant : Constant
  Constant1 : Constant  Value=N_Ind_M
  Constant2 : Constant  Value=3
  Logical Operator1 : Logic  Operator=NOT  AllPortsSameDT=off  OutDataTypeStr=boolean
  MinMax1 : MinMax  Inputs=2
  Product : Product  RndMeth=Zero
  Relational Operator : RelationalOperator  Operator=>  OutDataTypeStr=boolean  RndMeth=Nearest
  Sum : Sum  Inputs=|++
  Sum1 : Sum  Inputs=|++
  Unit Delay : UnitDelay  SampleTime=-1  HasFrameUpgradeWarning=on
  Enable : Outport
  Iteration : Outport  Port=2
  wires:
  Constant1/1 -> Sum1/1
  Constant2/1 -> Sum1/2
  Sum1/1 -> Product/1, Relational Operator/1
  Reset/1 -> Logical Operator1/1
  Logical Operator1/1 -> Product/2
  Relational Operator/1 -> Enable/1
  MinMax1/1 -> Relational Operator/2, Iteration/1, Unit Delay/1
  Unit Delay/1 -> Sum/2
  Sum/1 -> MinMax1/2
  Product/1 -> MinMax1/1
  Constant/1 -> Sum/1

== system Lib_Analytic/Numerical Methods/Jacobian Calculator/Jacobian ==
  Iteration : Inport
  Per : Inport  Port=2
  f(x_p) : Inport  Port=3
  Xo : Inport  Port=4
  Enable : EnablePort
  Jacobian Calc : MATLAB Function  TreatAsAtomicUnit=on
  Unit Delay : UnitDelay  InitialCondition=zeros(size(N_Per_M,2),size(N_Per_M,2))  SampleTime=-1  HasFrameUpgradeWarning=on
  Unit Delay1 : UnitDelay  InitialCondition=zeros(size(N_Per_M,2),prod(size(N_Per_M))+1)  SampleTime=-1  HasFrameUpgradeWarning=on
  Unit Delay2 : UnitDelay  InitialCondition=zeros(size(N_Per_M,2),1)  SampleTime=-1  HasFrameUpgradeWarning=on
  Unit Delay3 : UnitDelay  SampleTime=-1  HasFrameUpgradeWarning=on
  x_p : Outport
  Inv(J) : Outport  Port=2
  J : Outport  Port=3
  y_State : Outport  Port=4
  JacFailed : Outport  Port=5
  wires:
  Unit Delay3/1 -> Jacobian Calc/7(Er)
  Jacobian Calc/5(ErSv) -> JacFailed/1, Unit Delay3/1
  Unit Delay2/1 -> Jacobian Calc/2(y_xpIn)
  f(x_p)/1 -> Unit Delay2/1
  Unit Delay1/1 -> Jacobian Calc/6(y_StateIn)
  Jacobian Calc/4(y_StateOut) -> y_State/1, Unit Delay1/1
  Unit Delay/1 -> Jacobian Calc/5(JStateIn)
  Jacobian Calc/2(InvJOut) -> Inv(J)/1
  Jacobian Calc/3(JOut) -> J/1, Unit Delay/1
  Iteration/1 -> Jacobian Calc/1(IterationIn)
  Per/1 -> Jacobian Calc/3(PerIn)
  Xo/1 -> Jacobian Calc/4(XoIn)
  Jacobian Calc/1(XpOut) -> x_p/1

== system Lib_Analytic/Numerical Methods/Newton Raphson Solver/NR Update ==
  f(x) : Inport
  inv(J) : Inport  Port=2
  x(n) : Inport  Port=3
  Enable : EnablePort
  Bounding : Subsystem
  MatrixMult : Subsystem
  Sum : Sum  Inputs=|-+
  dxLimit : Subsystem
  x(n+1) : Outport
  wires:
  x(n)/1 -> Sum/2, dxLimit/2(x)
  Bounding/1(x(n+1)Lim) -> x(n+1)/1
  inv(J)/1 -> MatrixMult/2(inv(f'(x(n))))
  dxLimit/1(dx_limited) -> Sum/1
  MatrixMult/1(DTS) -> dxLimit/1(dx)
  Sum/1 -> Bounding/1(x(n+1)raw)
  f(x)/1 -> MatrixMult/1(f(x(n)))

== system Lib_Analytic/Solvers/Iterative NR Solver w JacobianCalc/JC w Reset ==
  note: Reset Jacobian Calculator after SJacobianAttempts_M
  f(x) : Inport  PortDimensions=length(SNR_IC_M)
  Iter : Inport  Port=2  PortDimensions=1
  x(n+1) : Inport  Port=3
  Enable : EnablePort
  Abs : Abs
  Constant : Constant  Value=SNR_IC_M
  Constant1 : Constant  Value=SJacobianAttempts_M  OutDataTypeStr=uint32
  Jacobian Calculator : Subsystem  TreatAsAtomicUnit=on  mask(T-MATS: Jacobian Calculator Library Block){N_Per_M=SJac_Per_M}
      mask prompts: N_Per_M "N_Per_M - Perturbations (nxm)"
      mask help:
      | The Jacobian Calculator block calculates the Jabobian of the system by perturbing the system around an initial point and calculating the gradient for each perturbation. This module will run once on start up and then again only if the reset is pressed.
      | Below: n (rows) is the number of times each independent will be perturbed and m (columns) is the number of inputs.
      mask Help: web(which('NumMthd_TMATS_JC.html'),'-helpbrowser')
  Product : Product  RndMeth=Zero
  Relational Operator : RelationalOperator  Operator===  OutDataTypeStr=boolean  RndMeth=Nearest
  Switch : Switch  Criteria=u2 ~= 0  Threshold=1
  Terminator3 : Terminator
  Unit Delay : UnitDelay  InitialCondition=SNR_IC_M./abs(SNR_IC_M)  SampleTime=-1  HasFrameUpgradeWarning=on
  J : Outport  PortDimensions=[length(SNR_IC_M),length(SNR_IC_M)]
  JacFailed : Outport  Port=2  PortDimensions=1
  X_out : Outport  Port=3  PortDimensions=length(SNR_IC_M)
  JC_Active : Outport  Port=4  PortDimensions=1
  inv(J) : Outport  Port=5  PortDimensions=[length(SNR_IC_M),length(SNR_IC_M)]
  wires:
  f(x)/1 -> Jacobian Calculator/2(f(x_p))
  Jacobian Calculator/5(inv(J)) -> inv(J)/1
  Unit Delay/1 -> Switch/3, Jacobian Calculator/3(Xo)
  x(n+1)/1 -> Unit Delay/1
  Jacobian Calculator/1(J) -> J/1  "J"
  Constant/1 -> Abs/1
  Relational Operator/1 -> Jacobian Calculator/1(Reset)
  Product/1 -> X_out/1
  Jacobian Calculator/2(x_p) -> Switch/1
  Switch/1 -> Product/1
  Jacobian Calculator/4(Active) -> Switch/2, JC_Active/1
  Constant1/1 -> Relational Operator/2
  Iter/1 -> Relational Operator/1
  Jacobian Calculator/3(Iteration) -> Terminator3/1
  Jacobian Calculator/6(JacFailed) -> JacFailed/1  "JacFalied"
  Abs/1 -> Product/2

== system Lib_Analytic/Solvers/Iterative NR Solver w JacobianCalc/NRwCond ==
  note: Enable NR when conditions are not met
      | and Jacobian Calculator is not active
  f(x) : Inport  PortDimensions=length(SNR_IC_M)
  JC_Active : Inport  Port=2  PortDimensions=1
  inv(f'(x)) : Inport  Port=3  PortDimensions=[length(SNR_IC_M),length(SNR_IC_M)]
  Enable : EnablePort
  Iteration Conditions : Subsystem
  Logical Operator : Logic  Operator=NOT  AllPortsSameDT=off  OutDataTypeStr=boolean
  Logical Operator1 : Logic  AllPortsSameDT=off  OutDataTypeStr=boolean
  Newton Raphson Solver : Subsystem  TreatAsAtomicUnit=on  mask(T-MATS: Newton Raphson Solver Library Block){NR_IC_M=SNR_IC_M./abs(SNR_IC_M), NR_dx_Lim_M=SNR_DX_M, NR_Mx_Lim_M=SNR_Mx_M./abs(SNR_IC_M), NR_Mn_Lim_M=SNR_Mn_M./abs(SNR_IC_M), BlkNm_M=double(gcb)}
      mask prompts: NR_IC_M "NR_IC_M - Initial Conditions of Newton Raphson (mx1)"; NR_dx_Lim_M "NR_dx_Lim_M - Newton Raphson step size limit (%) (1x1)"; NR_Mx_Lim_M "NR_Mx_Lim_M - Max limit (1x1 or mx1)"; NR_Mn_Lim_M "NR_Mn_Lim_M - Min Limit (1x1 or mx1)"; BlkNm_M "BlkNm_M - Block Name"
      mask help:
      | Newton Raphson Solver:
      |
      | x(n+1) = x(n) - inverse(f'(x(n)))*f(x(n))
      |
      | Note:
      | inverse(f'(x(n))) is an m x m matrix and f(x(n)) is an m x 1 matrix
      | where m is the length of the initial conditions matrix and number of system independents.
      mask init: same as Lib_Analytic/Numerical Methods/Newton Raphson Solver
      mask Help: web(which('NumMthd_TMATS_NRS.html'),'-helpbrowser')
  Terminator : Terminator
  CCnd : Outport  PortDimensions=1
  x(n+1) : Outport  Port=2  PortDimensions=length(SNR_IC_M)
  wires:
  f(x)/1 -> Newton Raphson Solver/3(f(x(n))), Iteration Conditions/1(f(x))
  JC_Active/1 -> Logical Operator/1
  Newton Raphson Solver/2(x(n+1)) -> x(n+1)/1
  Newton Raphson Solver/1(x(n)) -> Terminator/1
  inv(f'(x))/1 -> Newton Raphson Solver/2(inv(f'(x(n))))
  Logical Operator1/1 -> Newton Raphson Solver/1(Enable)
  Logical Operator/1 -> Logical Operator1/1
  Iteration Conditions/1(Condition) -> Logical Operator1/2, CCnd/1
